simulink model "PLANTAS_2"  (R2018a)
settings: Solver=ode4  StartTime=0.000001  StopTime=100  FixedStep=0.01  RelTol=1e-3
libraries: simulink x4
settings Model: Creator=ENIGMA  LastModifiedBy=root
settings CodeAppCC: StateflowObjectComments=on

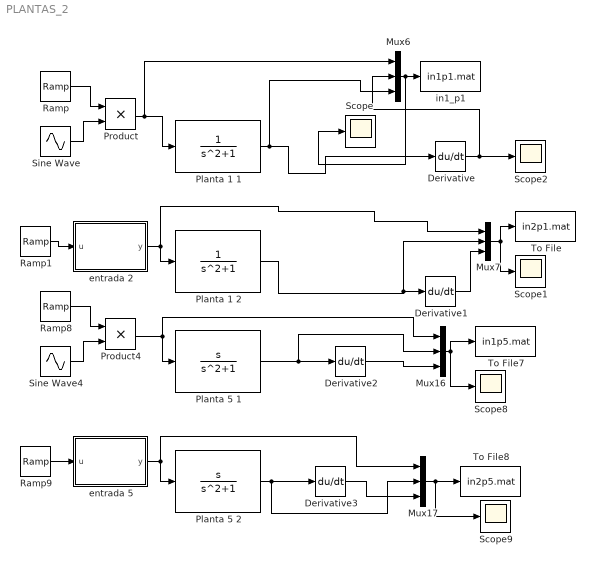
== system PLANTAS_2 ==
  Derivative{,1..3} (4 alike) : Derivative
  Mux{6..7,16..17} (4 alike) : Mux  Inputs=3
  Planta 1 1 : TransferFcn  Denominator=[1 0 1]
  Planta 1 2 : TransferFcn  Denominator=[1 0 1]
  Planta 5 1 : TransferFcn  Numerator=[1 0]  Denominator=[1 0 1]
  Planta 5 2 : TransferFcn  Numerator=[1 0]  Denominator=[1 0 1]
  Product : Product
  Product4 : Product
  Ramp : simulink/Sources/Ramp  slope=1  start=0  InitialOutput=0
  Ramp1 : simulink/Sources/Ramp  slope=1  start=0.0001  InitialOutput=0.0001
  Ramp8 : simulink/Sources/Ramp  slope=1  start=0  InitialOutput=0
  Ramp9 : simulink/Sources/Ramp  slope=1  start=0.0001  InitialOutput=0.0001
  Scope{,1..2,8..9} (5 alike) : Scope
  Sine Wave : Sin  Frequency=1/2  SampleTime=0
  Sine Wave4 : Sin  Frequency=1/2  SampleTime=0
  To File : ToFile  Filename=in2p1.mat  MatrixName=in2p1  SaveFormat=Timeseries
  To File7 : ToFile  Filename=in1p5.mat  MatrixName=in1p5
  To File8 : ToFile  Filename=in2p5.mat  MatrixName=in2p5  SaveFormat=Timeseries
  entrada 2 : MATLAB Function  TreatAsAtomicUnit=on
  entrada 5 : MATLAB Function  TreatAsAtomicUnit=on
  in1_p1 : ToFile  Filename=in1p1.mat  MatrixName=in1p1  SaveFormat=Timeseries
  wires:
  Planta 1 1/1 -> Derivative/1, Mux6/3
  Ramp/1 -> Product/1
  Sine Wave/1 -> Product/2
  Product/1 -> Mux6/1, Planta 1 1/1
  Planta 1 2/1 -> Derivative1/1, Mux7/2
  Ramp1/1 -> entrada 2/1(u)
  entrada 2/1(y) -> Planta 1 2/1, Mux7/1
  Mux6/1 -> Scope/1, in1_p1/1
  Mux7/1 -> To File/1, Scope1/1
  Planta 5 1/1 -> Derivative2/1, Mux16/2
  Ramp8/1 -> Product4/1
  Sine Wave4/1 -> Product4/2
  Product4/1 -> Mux16/1, Planta 5 1/1
  Planta 5 2/1 -> Mux17/2, Derivative3/1
  Ramp9/1 -> entrada 5/1(u)
  entrada 5/1(y) -> Planta 5 2/1, Mux17/1
  Mux16/1 -> To File7/1, Scope8/1
  Mux17/1 -> Scope9/1, To File8/1
  Derivative/1 -> Scope2/1, Mux6/2
  Derivative1/1 -> Mux7/3
  Derivative3/1 -> Mux17/3
  Derivative2/1 -> Mux16/3

== matlab function PLANTAS_2/entrada 2 ==
  data: u input; y output
function y = fcn(u)

y = (1/(u^1)) *sin ((u^10)/2);

== matlab function PLANTAS_2/entrada 5 ==
  data: u input; y output
function y = fcn(u)

y = (1/(u^1)) *sin ((u^10)/2);
